simulink model "LMS_cs_2018"  (R2018a)
settings: Solver=ode5  StartTime=0.0  StopTime=inf  FixedStep=1/200  RelTol=1e-3
PreLoadFcn:
  | mbxruntime.callbacks.PreLoadFcn(bdroot);
PostLoadFcn:
  | mbxruntime.callbacks.PostLoadFcn(bdroot);
InitFcn:
  | mbxruntime.callbacks.InitFcn(bdroot);
StartFcn:
  | mbxruntime.callbacks.StartFcn(bdroot);
StopFcn:
  | mbxruntime.callbacks.StopFcn(bdroot);
model workspace (MAT data in the model file):
  mbox_table : struct (value not decoded)
  model_closed = 0
  sim_status = 0
undefined symbols (not defined in the file or in its folder): DiscIntNeverNeededParam, serial, WheelL0, WheelL1, WheelR0, WheelR1
libraries: simulink x298, simulink_extras x78, PreScanSimulinkLibrary x29, PreScanUsefulBlocks x6, instrumentlib x5, simulink_need_slupdate x1
(part 2 of 45)

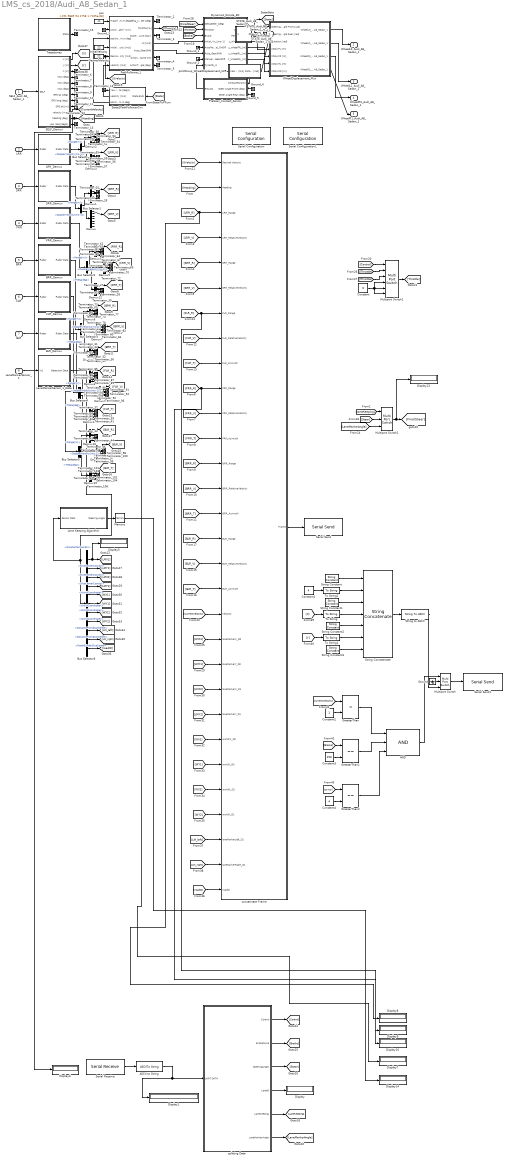
== system LMS_cs_2018/Audi_A8_Sedan_1 ==
  SELF_Audi_A8_Sedan_1 : Inport  Tag=inport/SelfPort  OutDataTypeStr=Bus: PRESCAN_SELFSENSORDATA  PortDimensions=1  SampleTime=2/200  BusOutputAsStruct=on
  LRR : Inport  Tag=inport/Radar  Port=2  OutDataTypeStr=Bus: PRESCAN_SCANNERSENSOR_MESSAGE  PortDimensions=7  SampleTime=1/4  BusOutputAsStruct=on
  SRR : Inport  Tag=inport/Radar  Port=3  OutDataTypeStr=Bus: PRESCAN_SCANNERSENSOR_MESSAGE  PortDimensions=7  SampleTime=1/4  BusOutputAsStruct=on
  FRR : Inport  Tag=inport/Radar  Port=4  OutDataTypeStr=Bus: PRESCAN_SCANNERSENSOR_MESSAGE  PortDimensions=7  SampleTime=1/4  BusOutputAsStruct=on
  BRR : Inport  Tag=inport/Radar  Port=5  OutDataTypeStr=Bus: PRESCAN_SCANNERSENSOR_MESSAGE  PortDimensions=7  SampleTime=1/4  BusOutputAsStruct=on
  FLR : Inport  Tag=inport/Radar  Port=6  OutDataTypeStr=Bus: PRESCAN_SCANNERSENSOR_MESSAGE  PortDimensions=7  SampleTime=1/4  BusOutputAsStruct=on
  BLR : Inport  Tag=inport/Radar  Port=7  OutDataTypeStr=Bus: PRESCAN_SCANNERSENSOR_MESSAGE  PortDimensions=7  SampleTime=1/4  BusOutputAsStruct=on
  LaneMarkerSensor_1 : Inport  Tag=inport/LaneMarker  Port=8  OutDataTypeStr=Bus: PRESCAN_LANEMARKER_MESSAGE  PortDimensions=2  SampleTime=1/20  BusOutputAsStruct=on
  AND : Logic  Inputs=3  IconShape=distinctive  AllPortsSameDT=off  OutDataTypeStr=boolean
  ASCII to String : ASCIIToString
  BLR_Demux : Subsystem  Tag=demux/Radar  TreatAsAtomicUnit=on  mask(PreScan Demux Block: Radar){MAXMESSAGES=7}
      mask prompts: MAXMESSAGES "Number of Objects"
      mask help:
      | The Radar Sensor is a detailed sensor based on a physical radar
      | model that includes Antenna GAIN Maps (AGM) and atmospheric
      | attenuation.
      |
      | For more information, please click Help.
      mask Help: eval('openHelp(1464)')
      mask Display:
      | port_label('input',1,'Radar')
      | port_label('output',1,'Radar Data')
  BRR_Demux : Subsystem  Tag=demux/Radar  TreatAsAtomicUnit=on  mask(PreScan Demux Block: Radar){MAXMESSAGES=7}
      mask prompts: MAXMESSAGES "Number of Objects"
      mask help:
      | The Radar Sensor is a detailed sensor based on a physical radar
      | model that includes Antenna GAIN Maps (AGM) and atmospheric
      | attenuation.
      |
      | For more information, please click Help.
      mask Help: eval('openHelp(1464)')
      mask Display:
      | port_label('input',1,'Radar')
      | port_label('output',1,'Radar Data')
  Bus Selector : BusSelector  OutputSignals=Range[m],DopplerVelocity[ms-1]
  Bus Selector1 : BusSelector  OutputSignals=Range[m],DopplerVelocity[ms-1]
  Bus Selector{2..5} (4 alike) : BusSelector  OutputSignals=Range[m],DopplerVelocity[ms-1],Theta[deg]
  Bus Selector6 : BusSelector  OutputSignals=ScanAtSensor.SliceCenterCoordsX,ScanAtSensor.SliceCenterCoordsY,ScanAtDistance1.SliceCenterCoordsX,ScanAtDistance1.SliceCenterCoordsY,ScanAtSensor.RightLaneIntersection1.WorldCoordinateX,ScanAtSensor.RightLaneIntersection1.WorldCoordinateY,ScanAtDistance1.RightLaneIntersection1.WorldCoordinateX,ScanAtDistance1.RightLaneIntersection1.WorldCoordinateY,ScanAtDistance1.LeftLaneIntersection1.DistanceFromScanCenter,ScanAtDistance1.RightLaneIntersection1.DistanceFromScanCenter,ScanAtDistance1.RoadIdUnderSliceCenter
  Constant : Constant  Value=0
  Constant1 : Constant  Value=4
  Constant2 : Constant
  Constant3 : Constant  Value=150
  Constant4 : Constant  Value=4
  Demux{,1..15} (16 alike) : Demux  Outputs=7
  DesiredVelocity : Constant  Tag=DesiredVelocity  Value=22
  Display{,1,5..10,13..14} (10 alike) : Display
  Dynamics_Simple_3D : Subsystem  Tag=Simple_Vehicle_Dynamics_3D  mask(PreScan Block: Simple Dynamics 3D){Migrate=on, TimeStep=1/200, ComputationMode=Continuous_Time}
      mask prompts: Migrate "Migrate. During migration this block will be replaced by a newer one."; TimeStep "Auto assigned: Time Step [s]"; ComputationMode "Computation mode:"
      mask help:
      | The Simple Dynamics Model is selected in the GUI to simulate vehicle dynamics behavior.
      |
      | The Simple Dynamics Model is completely open to the user. The parameters of this model can be set in the Simple Dynamics dialog in the GUI.
      |
      | For more information, please click Help.
      mask init:
      | p = SimpleDyn_pars;
      settings: DeleteFcn=PreScanBlockDeleteFcn;
      mask Help: eval('openHelp(260)')
      mask Display:
      | image(imread('SimpleDyn.png'))
      | port_label('input', 1, '{\delta}_S_t_ _e_e_r [deg]','texmode','on')
      | port_label('input', 2, 'Throttle [%]')
      | port_label('input', 3, 'Brake Pres [bar]')
      | port_label('input', 4, 'V_0 [ms-1]','texmode','on')
      | port_label('input', 5, 'Auto=[0]/Manual=[1]')
      | port_label('input', 6, 'Auto_GearShift')
      | port_label('input', 7, 'Manual_GearShift')
      | port_label('input', 8, 'TyreInfo_in')
      | port_label('output', 1, 'State')
      | port_label('output', 2, 'Vx [ms-1]')
      | port_label('output', 3, 'Perf Params')
      | port_label('output', 4, 'zDispFL[m]')
      | port_label('output', 5, 'zDispFR[m]')
      | port_label('output', 6, 'zDispRL[m]')
      | port_label('output', 7, 'zDispRR[m]')
  FLR_Demux : Subsystem  Tag=demux/Radar  TreatAsAtomicUnit=on  mask(PreScan Demux Block: Radar){MAXMESSAGES=7}
      mask prompts: MAXMESSAGES "Number of Objects"
      mask help:
      | The Radar Sensor is a detailed sensor based on a physical radar
      | model that includes Antenna GAIN Maps (AGM) and atmospheric
      | attenuation.
      |
      | For more information, please click Help.
      mask Help: eval('openHelp(1464)')
      mask Display:
      | port_label('input',1,'Radar')
      | port_label('output',1,'Radar Data')
  FRR_Demux : Subsystem  Tag=demux/Radar  TreatAsAtomicUnit=on  mask(PreScan Demux Block: Radar){MAXMESSAGES=7}
      mask prompts: MAXMESSAGES "Number of Objects"
      mask help:
      | The Radar Sensor is a detailed sensor based on a physical radar
      | model that includes Antenna GAIN Maps (AGM) and atmospheric
      | attenuation.
      |
      | For more information, please click Help.
      mask Help: eval('openHelp(1464)')
      mask Display:
      | port_label('input',1,'Radar')
      | port_label('output',1,'Radar Data')
  GreaterThan : RelationalOperator  Operator=<  OutDataTypeStr=boolean  RndMeth=Simplest
  GreaterThan1 : RelationalOperator  Operator===  OutDataTypeStr=boolean  RndMeth=Simplest
  GreaterThan2 : RelationalOperator  Operator===  OutDataTypeStr=boolean  RndMeth=Simplest
  Ground : Ground
  Ground_{1..7} (7 alike) : Ground
  InitialVelocity : Constant  Tag=InitialVelocity  Value=22
  JointGroup_WheelDisplacement_V2R : Subsystem  Tag=mux/Wheels  mask(PreScan Velocity to Wheel Angle Block:){TimeStep=2/200, TireRadius=0.34}
      mask prompts: TimeStep "Auto Assigned: Time Step [s]"; TireRadius "Tire Radius [m]"
      settings: DeleteFcn=PreScanBlockDeleteFcn;
      mask Display: disp('Velocity\nto\nWheelAngle')
  LRR_Demux : Subsystem  Tag=demux/Radar  TreatAsAtomicUnit=on  mask(PreScan Demux Block: Radar){MAXMESSAGES=7}
      mask prompts: MAXMESSAGES "Number of Objects"
      mask help:
      | The Radar Sensor is a detailed sensor based on a physical radar
      | model that includes Antenna GAIN Maps (AGM) and atmospheric
      | attenuation.
      |
      | For more information, please click Help.
      mask Help: eval('openHelp(1464)')
      mask Display:
      | port_label('input',1,'Radar')
      | port_label('output',1,'Radar Data')
  Lane Keeping Algorithm : Subsystem
  LaneMarkerSensor_1_Data : Subsystem  Tag=demux/LaneMarkerSensor  mask{NUMBEROFSLICES=2, TimeStep=1/20}
      mask prompts: NUMBEROFSLICES "Number of slices"; TimeStep "Auto Assigned: Time Step [s]"
      mask Help: eval('openHelp(2301)')
  Memory : Memory
  Multiport Switch : MultiPortSwitch  DataPortOrder=Zero-based contiguous  Inputs=2  zeroidx=on
  Multiport Switch1 : MultiPortSwitch  DataPortOrder=Zero-based contiguous  Inputs=5  zeroidx=on
  Multiport Switch2 : MultiPortSwitch  DataPortOrder=Zero-based contiguous  Inputs=2  zeroidx=on
  PathFollower_1 : Subsystem  Tag=pathFollower  mask(PreScan Block: Path Follower){Migrate=on, FileName='Trajectory_1.mat', TunableSteeringGain=1, XShifting_wrt_COG=0}
      mask prompts: Migrate "Migrate. During migration this block will be replaced by a newer one."; FileName "Trajectory Name"; TunableSteeringGain "TunableSteeringGain [-]"; XShifting_wrt_COG "XShifting_wrt_COG [m]"
      mask help:
      | The Path Follower Model is selected in the GUI to simulate driver behavior.
      |
      | For more information, please click Help.
      mask init:
      | load(['trajectories/',eval(FileName)])
      | traject=trajectory';
      | 
      | Traj_x=traject(:,2);
      | Traj_y=traject(:,3);
      | Traj_z=traject(:,4);
      | Traj_vx=traject(:,8);
      | Traj_vy=traject(:,9);
      | Traj_vz=traject(:,10);
      mask Help: eval('openHelp(232)')
  PreScan_Contact_Sensor : Subsystem  Tag=PreScan_Contact_Sensor  LoadFcn=|  mask(PreScan Block: PreScan Contact Sensor){x0=-191.9885, y0=94.1758, z0=0.55, Roll0=0, Pitch0=0, Yaw0=1.7105e-08, wheelRadius=0.34, hcog=0.55, b=1.77, TimeStep=1/200}
      | load PrescanXYZData;
      | load PrescanRPYData;
      | load PrescanQuatData;
      | load PrescanAxisAngleData;
      | load PrescanPoseData;
      | load PrescanPoseQData;
      | load PrescanPoseAData;
      | load PrescanWheelContactData;
      mask prompts: x0 "Ini x-position VEHICLE wrt GLOBAL axis system [m]"; y0 "Ini y-position VEHICLE wrt GLOBAL axis system [m]"; z0 "Ini z-position VEHICLE wrt GLOBAL axis system [m]"; Roll0 "Ini roll-angle BODY wrt VEHICLE axis system [deg]"; Pitch0 "Ini pitch-angle BODY wrt VEHICLE axis system [deg]"; Yaw0 "Ini yaw-angle VEHICLE wrt GLOBAL axis system [deg]"; wheelRadius "Wheel Radius [m]"; hcog "Dynamics: hCoG [m]"; b "Dynamics: b [m]"; TimeStep "Time Step [s]"
      mask help:
      | This block encapsulates the base Contact sensor.
      |
      | It takes input parameters from the PreScan 3D vehicle dynamics block and outputs contact results.
      mask Help: eval('openHelp(251)')
  SELF_Demux : Subsystem  Tag=demux/SelfPort  mask(PreScan Demux Block:){}
      mask help:
      | The SELF port shows (state) information of the actor itself. The outputs are position in the experiment's axis system and the GPS coordinates, and the object's absolute velocity and compass heading.
      |
      | For more information, please click Help.
      settings: DeleteFcn=PreScanBlockDeleteFcn;
      mask Help: eval('openHelp(462)')
      mask Display:
      | port_label('output',1,'x [m]')
      | port_label('output',2,'y [m]')
      | port_label('output',3,'z [m]','texmode','on')
      | port_label('output',4,'Rotx [deg]','texmode','on')
      | port_label('output',5,'Roty [deg]','texmode','on')
      | port_label('output',6,'Rotz [deg]','texmode','on')
      | port_label('output',7,'GPS lat [deg]','texmode','on')
      | port_label('output',8,'GPS long [deg]','texmode','on')
      | port_label('output',9,'GPS alt [m]','texmode','on')
      | port_label('output',10,'Velocity [m/s]')
      | port_label('output',11,'Heading [deg]')
      | port_label('output',12,'Yaw rate [deg/s]')
  SRR_Demux : Subsystem  Tag=demux/Radar  TreatAsAtomicUnit=on  mask(PreScan Demux Block: Radar){MAXMESSAGES=7}
      mask prompts: MAXMESSAGES "Number of Objects"
      mask help:
      | The Radar Sensor is a detailed sensor based on a physical radar
      | model that includes Antenna GAIN Maps (AGM) and atmospheric
      | attenuation.
      |
      | For more information, please click Help.
      mask Help: eval('openHelp(1464)')
      mask Display:
      | port_label('input',1,'Radar')
      | port_label('output',1,'Radar Data')
  STATE_Audi_A8_Sedan_1 : Subsystem  Tag=mux/StatePort  Priority=0  LoadFcn=load PrescanStateActuatorData  mask(PreScan Sink Block: State){x0=-191.9885, y0=94.1758, z0=0.55, Roll0=0, Pitch0=0, Yaw0=1.7105e-08, TimeStep=1/200}
      mask prompts: x0 "Ini x-position VEHICLE wrt GLOBAL axis system [m]"; y0 "Ini y-position VEHICLE wrt GLOBAL axis system [m]"; z0 "Ini z-position VEHICLE wrt GLOBAL axis system [m]"; Roll0 "Ini roll-angle BODY wrt VEHICLE axis system [deg]"; Pitch0 "Ini pitch-angle BODY wrt VEHICLE axis system [deg]"; Yaw0 "Ini yaw-angle VEHICLE wrt GLOBAL axis system [deg]"; TimeStep "Auto-Assigned: Upload Period [s]"
      mask help:
      | The Actor State contains a vector signal of size (9x1), containing the following signals:
      |
      | -  Position                  (x,y,z)                                     [m]
      | -  Velocity                  (vx,vy,vz)                               [m/s]
      | -  Angles                    (Roll, Pitch, Yaw)                   [rad]
      |
      | The Actor state is defined in the global axis system.
      | The state is superponed on the Initial position defined in the GUI.
      |
      | For more information, please click Help.
      settings: DeleteFcn=PreScanBlockDeleteFcn;
      mask Help: eval('openHelp(222)')
      mask Display: image(imread('State.png'))
  STATE_Audi_A8_Sedan_1_rc : RateTransition  Tag=mux_rc/StatePort  OutPortSampleTimeOpt=Inherit
  Serial Receive : instrumentlib/Serial Receive  Priority=1  ObjConstructor=serial('COM5');  ComPortMenu=COM5  ComPort=COM5  DataType=uint8  DataSize="[1  21]"  EnableBlockingMode=on  ActionDataUnavailable=Output last received value  CustomValue=0  SampleTime=0.005
  Serial Configuration : instrumentlib/Serial Configuration  Priority=-200000  ObjConstructor=serial('COM5');  ComPortMenu=COM5  ComPort=COM5  BaudRate=115200  DataBits=8  Parity=none  StopBits=1  ByteOrder=LittleEndian  FlowControl=none  Timeout=0.001
  Serial Configuration1 : instrumentlib/Serial Configuration  Priority=-200000  PortSel=COM6  Port=COM6  ComPort=COM6  BaudRate=115200  DataBits=8  Parity=none  StopBits=1  ByteOrder=little-endian  FlowControl=none  Timeout=0.001  SimulateUsing=Interpreted execution  BlockInModel=on  aMode=1
  Serial Send : instrumentlib/Serial Send  Priority=1  ObjConstructor=serial('COM5');  ComPortMenu=COM5  ComPort=COM5  Terminator=<none>  EnableBlockingMode=on
  Serial Send1 : instrumentlib/Serial Send  Priority=1  PortSel=COM6  Port=COM6  ComPort=COM6  Header=[]  Terminator=<none>  CustomTerminator=[]  EnableBlockingMode=on  SimulateUsing=Interpreted execution  BlockInModel=on  aMode=1
  State2PathFollowerCnv : Subsystem  Tag=State2PFConnection/cnv
  String Concatenate : StringConcatenate  Inputs=7
  String Constant : StringConstant  String="\"*\""
  String Constant1 : StringConstant  String="\";\""
  String Constant2 : StringConstant  String="\"/\""
  String Constant3 : StringConstant  String="\"#\""
  String to ASCII : StringToASCII  MaximumLength=30
  Terminator_{1..15,24..106} (98 alike) : Terminator
  To String : ToString
  To String1 : ToString
  To String2 : ToString
  Trajectories : Subsystem  Tag=Trajectories  mask(PreScan Source Block: Trajectories){}
      mask help:
      | The Trajectory block contains the trajectories defined in the PreScan Experiment Editor. The output of the trajectory block is the (vehicle) State.
      |
      | For more information, please click Help.
      settings: DeleteFcn=PreScanBlockDeleteFcn;
      mask Help: eval('openHelp(312)')
      mask Display: image(imread('Trajectory.png'));
  WheelDisplacement_Mux : Subsystem  Tag=mux/JointGroup  mask(JointGroup){}
      mask help:
      | The JointGroup allows to control several Joints in one go, as defined for this particular model.
      | For more information, look in the PreScan manual in the section "Model Preparation Tool" -> "Joint Groups"
      |
      | For more information on the Joints simulink interface, press Help.
      mask Help: eval('openHelp(254)')
  concatinate Frame : Subsystem
  pos : Constant  Tag=pos  Value=[-191.9885 94.1758 1.7105e-08]
  splitting Data : Subsystem
  STATE_Audi_A8_Sedan_1_bus : Outport  Tag=outport/StatePort  OutDataTypeStr=Bus: PRESCAN_STATEACTUATORDATA  PortDimensions=1  SampleTime=2/200
  WheelL0_Audi_A8_Sedan_1 : Outport  Tag=outport/JointActuator  Port=2  OutDataTypeStr=Bus: PRESCAN_POSE_DATA  SampleTime=2/200
  WheelL1_Audi_A8_Sedan_1 : Outport  Tag=outport/JointActuator  Port=3  OutDataTypeStr=Bus: PRESCAN_POSE_DATA  SampleTime=2/200
  WheelR0_Audi_A8_Sedan_1 : Outport  Tag=outport/JointActuator  Port=4  OutDataTypeStr=Bus: PRESCAN_POSE_DATA  SampleTime=2/200
  WheelR1_Audi_A8_Sedan_1 : Outport  Tag=outport/JointActuator  Port=5  OutDataTypeStr=Bus: PRESCAN_POSE_DATA  SampleTime=2/200
  wires:
  Lane Keeping Algorithm/1(Steering Angle) -> Memory/1
  Demux2/5 -> Terminator_52/1
  Bus Selector/1 -> Demux2/1  "<Range[m]>"
  Demux3/4 -> Terminator_57/1
  Demux2/7 -> Terminator_54/1
  Demux2/4 -> Terminator_51/1
  Demux3/6 -> Terminator_59/1
  Demux3/7 -> Terminator_60/1
  Demux3/3 -> Terminator_56/1
  Demux2/3 -> Terminator_50/1
  Demux2/2 -> Terminator_49/1
  Demux2/6 -> Terminator_53/1
  Demux2/1 -> [LRR_R]
  Bus Selector/2 -> Demux3/1  "<DopplerVelocity[ms-1]>"
  Demux3/1 -> [LRR_V]
  Demux3/5 -> Terminator_58/1
  Demux3/2 -> Terminator_55/1
  LRR_Demux/1(Radar Data) -> Bus Selector/1
  Demux/3 -> ?
  Demux/2 -> ?
  Demux/4 -> ?
  Demux/5 -> ?
  Demux/6 -> ?
  Demux/7 -> ?
  Demux1/2 -> ?
  Demux1/4 -> Terminator_26/1
  Demux1/7 -> Terminator_24/1
  Bus Selector1/1 -> Demux1/1  "<Range[m]>"
  Bus Selector1/2 -> Demux/1  "<DopplerVelocity[ms-1]>"
  Demux1/3 -> Terminator_25/1
  Demux/1 -> [SRR_V]
  Demux1/1 -> [SRR_R]
  Demux1/6 -> ?
  Demux1/5 -> ?
  SRR_Demux/1(Radar Data) -> Bus Selector1/1
  Demux12/4 -> Terminator_27/1
  Demux4/2 -> Terminator_61/1
  Demux5/2 -> Terminator_67/1
  Demux12/6 -> Terminator_29/1
  Demux4/6 -> Terminator_65/1
  Demux5/5 -> Terminator_70/1
  Demux12/2 -> ?
  Demux5/6 -> Terminator_71/1
  Demux5/4 -> Terminator_69/1
  Demux4/1 -> [FRR_R]
  Demux4/4 -> Terminator_63/1
  Demux4/7 -> Terminator_66/1
  Demux12/1 -> [FRR_T]
  Demux4/3 -> Terminator_62/1
  Demux12/7 -> Terminator_30/1
  Demux4/5 -> Terminator_64/1
  Demux12/3 -> ?
  Demux5/7 -> Terminator_72/1
  Demux5/3 -> Terminator_68/1
  Demux5/1 -> [FRR_V]
  Demux12/5 -> Terminator_28/1
  Bus Selector2/3 -> Demux12/1  "<Theta[deg]>"
  Bus Selector2/1 -> Demux4/1  "<Range[m]>"
  Bus Selector2/2 -> Demux5/1  "<DopplerVelocity[ms-1]>"
  FRR_Demux/1(Radar Data) -> Bus Selector2/1
  Demux13/4 -> Terminator_33/1
  Bus Selector3/3 -> Demux13/1  "<Theta[deg]>"
  Demux7/7 -> Terminator_84/1
  Demux13/5 -> Terminator_34/1
  Demux7/3 -> Terminator_80/1
  Demux6/3 -> Terminator_74/1
  Demux13/3 -> Terminator_32/1
  Demux7/6 -> Terminator_83/1
  Demux6/2 -> Terminator_73/1
  Demux7/4 -> Terminator_81/1
  Demux7/5 -> Terminator_82/1
  Demux7/2 -> Terminator_79/1
  Demux6/4 -> Terminator_75/1
  Demux6/6 -> Terminator_77/1
  Demux6/5 -> Terminator_76/1
  Demux6/1 -> [BRR_R]
  Demux7/1 -> [BRR_V]
  Bus Selector3/1 -> Demux6/1  "<Range[m]>"
  Demux13/6 -> Terminator_35/1
  Bus Selector3/2 -> Demux7/1  "<DopplerVelocity[ms-1]>"
  Demux13/2 -> Terminator_31/1
  Demux13/7 -> Terminator_36/1
  Demux6/7 -> Terminator_78/1
  Demux13/1 -> [BRR_T]
  BRR_Demux/1(Radar Data) -> Bus Selector3/1
  Demux14/4 -> Terminator_39/1
  Demux14/5 -> Terminator_40/1
  Bus Selector4/2 -> Demux9/1  "<DopplerVelocity[ms-1]>"
  Demux9/7 -> Terminator_96/1
  Demux8/3 -> Terminator_86/1
  Demux8/5 -> Terminator_88/1
  Demux9/4 -> Terminator_93/1
  Demux8/6 -> Terminator_89/1
  Demux8/4 -> Terminator_87/1
  Demux8/7 -> Terminator_90/1
  Demux8/2 -> Terminator_85/1
  Demux8/1 -> [FLR_R]
  Demux14/2 -> Terminator_37/1
  Demux14/6 -> Terminator_41/1
  Demux9/3 -> Terminator_92/1
  Demux9/2 -> Terminator_91/1
  Demux9/1 -> [FLR_V]
  Demux9/5 -> Terminator_94/1
  Demux14/3 -> Terminator_38/1
  Bus Selector4/1 -> Demux8/1  "<Range[m]>"
  Demux9/6 -> Terminator_95/1
  Bus Selector4/3 -> Demux14/1  "<Theta[deg]>"
  Demux14/7 -> Terminator_42/1
  Demux14/1 -> [FLR_T]
  FLR_Demux/1(Radar Data) -> Bus Selector4/1
  Demux15/6 -> Terminator_105/1
  Demux15/3 -> Terminator_102/1
  Demux15/1 -> [BLR_T]
  Demux10/3 -> ?
  Demux15/2 -> Terminator_101/1
  Demux11/2 -> Terminator_47/1
  Demux11/7 -> Terminator_100/1
  Demux11/5 -> Terminator_98/1
  Demux11/6 -> Terminator_99/1
  Demux11/4 -> Terminator_97/1
  Demux15/5 -> Terminator_104/1
  Demux15/4 -> Terminator_103/1
  Demux10/4 -> Terminator_43/1
  Demux10/2 -> ?
  Demux11/3 -> Terminator_48/1
  Bus Selector5/1 -> Demux10/1  "<Range[m]>"
  Demux15/7 -> Terminator_106/1
  Demux10/1 -> [BLR_R]
  Demux10/6 -> Terminator_45/1
  Demux11/1 -> [BLR_V]
  Bus Selector5/2 -> Demux11/1  "<DopplerVelocity[ms-1]>"
  Bus Selector5/3 -> Demux15/1  "<Theta[deg]>"
  Demux10/7 -> Terminator_46/1
  Demux10/5 -> Terminator_44/1
  BLR_Demux/1(Radar Data) -> Bus Selector5/1
  [FLR_R] -> Display10/1, concatinate Frame/7(" FLR_Range")
  [SRR_R] -> concatinate Frame/5(" SRR_Range")
  [LRR_V] -> concatinate Frame/4(LRR_RelativeVelocity)
  [BLR_T] -> concatinate Frame/18(" BLR_Azimuth")
  [FRR_R] -> Display9/1, concatinate Frame/10(" FRR_Range")
  [BRR_T] -> concatinate Frame/15(" BRR_Azimuth")
  [FLR_T] -> concatinate Frame/9(FLR_Azimuth)
  [FRR_T] -> concatinate Frame/12(" FRR_Azimuth")
  [FRR_V] -> concatinate Frame/11(" FRR_RelativeVelocity")
  [LRR_R] -> Display8/1, concatinate Frame/3(" LRR_Range")
  [FLR_V] -> concatinate Frame/8(" FLR_RelativeVelocity")
  concatinate Frame/1(Frame) -> Serial Send/1
  [BLR_V] -> concatinate Frame/17(" BLR_RelativeVelocity")
  [BRR_V] -> concatinate Frame/14(" BRR_RelativeVelocity")
  [SRR_V] -> concatinate Frame/6(" SRR_RelativeVelocity")
  [BLR_R] -> concatinate Frame/16(" BLR_Range")
  [Heading] -> concatinate Frame/2(Heading)
  [BRR_R] -> concatinate Frame/13(" BRR_Range")
  splitting Data/1(Control) -> [Control]
  Serial Receive/1 -> ASCII to String/1
  ASCII to String/1 -> splitting Data/1(UART DATA), Display1/1
  splitting Data/2(BrakeForce) -> [Brake]
  splitting Data/4(LaneID) -> Display/1
  splitting Data/3(SteeringAngle) -> [Steer]
  Constant/1 -> Multiport Switch1/6, Multiport Switch1/4, Multiport Switch1/5
  [IThrottle] -> Multiport Switch1/3
  [Control] -> Multiport Switch1/1
  [IThrottle] -> Multiport Switch1/2
  Multiport Switch1/1 -> [Throttle]
  SELF_Demux/11(heading [deg]) -> Display7/1, [Heading]
  PathFollower_1/2(throttle [%]) -> [IThrottle]
  [Throttle] -> Dynamics_Simple_3D/2(Throttle)
  [Brake] -> Dynamics_Simple_3D/3(Brake)
  PathFollower_1/4(v0 [m/s]) -> Dynamics_Simple_3D/4(Initial_Vx_[ms-1])
  Multiport Switch2/1 -> Display13/1, [FinalSteer]
  SELF_Demux/10(velocity [m/s]) -> Display6/1, [CurrentVelocity]
  [FinalSteer] -> Dynamics_Simple_3D/1(DeltaSteer_[deg])
  [LaneKeeping] -> Multiport Switch2/1
  [Steer] -> Multiport Switch2/2
  splitting Data/5(LaneKeeping) -> [LaneKeeping]
  [DVelocity] -> concatinate Frame/1(" Desired Velocity")
  [CurrentVelocity] -> concatinate Frame/19(Velocity)
  splitting Data/6(LaneMarkerAngle) -> [LaneMarkerAngle]
  LaneMarkerSensor_1_Data/1(Detection Data) -> Bus Selector6/1, Lane Keeping Algorithm/1(Sensor Data)
  Bus Selector6/1 -> Display5/1, [LMX1]  "<SliceCenterCoordsX>"
  Bus Selector6/2 -> [LMY1]  "<SliceCenterCoordsY>"
  Bus Selector6/3 -> [LMX2]  "<SliceCenterCoordsX>"
  Bus Selector6/4 -> [LMY2]  "<SliceCenterCoordsY>"
  Bus Selector6/5 -> [WX1]  "<WorldCoordinateX>"
  Bus Selector6/6 -> [WY1]  "<WorldCoordinateY>"
  Bus Selector6/7 -> [WX2]  "<WorldCoordinateX>"
  Bus Selector6/8 -> [WY2]  "<WorldCoordinateY>"
  Bus Selector6/11 -> [roadID]  "<RoadIdUnderSliceCenter>"
  [LMX1] -> concatinate Frame/20(laneMarkerX_D0)
  [LMY1] -> concatinate Frame/21(laneMarkerY_D0)
  [LMX2] -> concatinate Frame/22(laneMarkerX_D1)
  [LMY2] -> concatinate Frame/23(laneMarkerY_D1)
  [WX2] -> concatinate Frame/26(worldX_D1)
  [WY1] -> concatinate Frame/25(worldY_D0)
  [WX1] -> concatinate Frame/24(worldrX_D0)
  [WY2] -> concatinate Frame/27(worldY_D1)
  [roadID] -> concatinate Frame/30(roadID)
  [LM_left] -> concatinate Frame/28(laneMarkerLeft_D1)
  [LM_right] -> concatinate Frame/29(laneMarkerRight_D1)
  Bus Selector6/9 -> [LM_left]  "<DistanceFromScanCenter>"
  Bus Selector6/10 -> [LM_right]  "<DistanceFromScanCenter>"
  Memory/1 -> Display14/1
  [LaneMarkerAngle] -> Multiport Switch2/3
  DesiredVelocity/1 -> [DVelocity], PathFollower_1/5(Desired Velocity [m/s])
  SELF_Demux/1(x [m]) -> [X]
  SELF_Demux/2(y [m]) -> [Y]
  [X] -> To String/1
  [Y] -> To String1/1
  Constant1/1 -> To String2/1
  To String2/1 -> String Concatenate/2
  To String/1 -> String Concatenate/4
  To String1/1 -> String Concatenate/6
  String Constant/1 -> String Concatenate/1
  String Constant1/1 -> String Concatenate/3
  String Constant2/1 -> String Concatenate/5
  String Constant3/1 -> String Concatenate/7
  String Concatenate/1 -> String to ASCII/1
  STATE_Audi_A8_Sedan_1_rc/1 -> STATE_Audi_A8_Sedan_1_bus/1
  STATE_Audi_A8_Sedan_1/1(StateBus) -> STATE_Audi_A8_Sedan_1_rc/1, [State]
  SELF_Audi_A8_Sedan_1/1 -> SELF_Demux/1(SELF)
  LRR/1 -> LRR_Demux/1(Radar)
  SRR/1 -> SRR_Demux/1(Radar)
  FRR/1 -> FRR_Demux/1(Radar)
  BRR/1 -> BRR_Demux/1(Radar)
  FLR/1 -> FLR_Demux/1(Radar)
  BLR/1 -> BLR_Demux/1(Radar)
  LaneMarkerSensor_1/1 -> LaneMarkerSensor_1_Data/1(In1)
  WheelDisplacement_Mux/1(WheelL0_Audi_A8_Sedan_1) -> WheelL0_Audi_A8_Sedan_1/1
  WheelDisplacement_Mux/2(WheelL1_Audi_A8_Sedan_1) -> WheelL1_Audi_A8_Sedan_1/1
  WheelDisplacement_Mux/3(WheelR0_Audi_A8_Sedan_1) -> WheelR0_Audi_A8_Sedan_1/1
  WheelDisplacement_Mux/4(WheelR1_Audi_A8_Sedan_1) -> WheelR1_Audi_A8_Sedan_1/1
  JointGroup_WheelDisplacement_V2R/1(Rotation [rad]) -> WheelDisplacement_Mux/3(Rotation [rad])
  Dynamics_Simple_3D/8(ContactParams) -> PreScan_Contact_Sensor/1(ContactParams)
  PreScan_Contact_Sensor/1(Results) -> Dynamics_Simple_3D/8(TyreInfo_in)
  Dynamics_Simple_3D/2(Vx [m s-1]) -> JointGroup_WheelDisplacement_V2R/1(Velocity [m/s])
  Dynamics_Simple_3D/4(z_wheelFL_[m]) -> WheelDisplacement_Mux/4(zDisp FL [m])
  Dynamics_Simple_3D/5(z_wheelFR_[m]) -> WheelDisplacement_Mux/5(zDisp FR [m])
  Dynamics_Simple_3D/6(z_wheelRL_[m]) -> WheelDisplacement_Mux/6(zDisp RL [m])
  Dynamics_Simple_3D/7(z_wheelRR_[m]) -> WheelDisplacement_Mux/7(zDisp RR [m])
  pos/1 -> PathFollower_1/1(TrajOffset_x,y,Y [m,m,deg])
  InitialVelocity/1 -> PathFollower_1/4(Initial Velocity [m/s])
  [State] -> State2PathFollowerCnv/1(State BUS)
  State2PathFollowerCnv/2(velocity [m/s]) -> PathFollower_1/6(velocity [m/s])
  State2PathFollowerCnv/3(position x,y,Y [m,m,deg]) -> PathFollower_1/3(position x,y,Y [m,m,deg])
  PathFollower_1/5(Auto_GearShift) -> Dynamics_Simple_3D/6(Auto_GearShift)
  Dynamics_Simple_3D/1(State) -> STATE_Audi_A8_Sedan_1/1(State)
  Ground_1/1 -> Dynamics_Simple_3D/5(AutoManual_OnOff)
  Ground_2/1 -> Dynamics_Simple_3D/7(Manual_GearShift)
  Dynamics_Simple_3D/3(Perf_Params) -> Terminator_1/1
  Ground_3/1 -> PathFollower_1/2(ActorOffset_Left(+) / Right(-) [m])
  PathFollower_1/1(delta_steerwheel [deg]) -> Terminator_2/1
  PathFollower_1/3(brake pressure [bar]) -> Terminator_3/1
  PathFollower_1/6(Actor/Traj_distance [m]) -> Terminator_4/1
  PathFollower_1/7(Actor/Traj_angle [deg]) -> Terminator_5/1
  Ground_4/1 -> PreScan_Contact_Sensor/2(Steer Angle Front [deg])
  Ground_5/1 -> PreScan_Contact_Sensor/3(Steer Angle Rear [deg])
  SELF_Demux/3(z [m]) -> Terminator_6/1
  SELF_Demux/4(rotx [deg]) -> Terminator_7/1
  SELF_Demux/5(roty [deg]) -> Terminator_8/1
  SELF_Demux/6(rotz [deg]) -> Terminator_9/1
  SELF_Demux/7(GPS lat [deg]) -> Terminator_10/1
  SELF_Demux/8(GPS long [deg]) -> Terminator_11/1
  SELF_Demux/9(GPS alt [m]) -> Terminator_12/1
  SELF_Demux/12(yaw rate [deg/s]) -> Terminator_13/1
  State2PathFollowerCnv/1(Yaw rate [deg/s]) -> Terminator_14/1
  Trajectories/1(State) -> Terminator_15/1
  Ground_6/1 -> WheelDisplacement_Mux/1(Steering Angle Front [rad])
  Ground_7/1 -> WheelDisplacement_Mux/2(Steering Angle Rear [rad])
  Constant2/1 -> GreaterThan/2
  [CurrentVelocity] -> GreaterThan/1
  GreaterThan/1 -> AND/1
  Constant3/1 -> GreaterThan1/2
  [Brake] -> GreaterThan1/1
  GreaterThan1/1 -> AND/2
  Multiport Switch/1 -> Serial Send1/1
  AND/1 -> Multiport Switch/1
  String to ASCII/1 -> Multiport Switch/3
  Ground/1 -> Multiport Switch/2
  [Control] -> GreaterThan2/1
  Constant4/1 -> GreaterThan2/2
  GreaterThan2/1 -> AND/3

== system LMS_cs_2018/Audi_A8_Sedan_2 ==
  SELF_Audi_A8_Sedan_2 : Inport  Tag=inport/SelfPort  OutDataTypeStr=Bus: PRESCAN_SELFSENSORDATA  PortDimensions=1  SampleTime=2/200  BusOutputAsStruct=on
  Auto_Gear : Constant  Tag=AutoGear
  Dynamics_Simple_3D : Subsystem  Tag=Simple_Vehicle_Dynamics_3D  mask(PreScan Block: Simple Dynamics 3D){Migrate=on, TimeStep=1/200, ComputationMode=Continuous_Time}
      mask prompts: Migrate "Migrate. During migration this block will be replaced by a newer one."; TimeStep "Auto assigned: Time Step [s]"; ComputationMode "Computation mode:"
      mask help:
      | The Simple Dynamics Model is selected in the GUI to simulate vehicle dynamics behavior.
      |
      | The Simple Dynamics Model is completely open to the user. The parameters of this model can be set in the Simple Dynamics dialog in the GUI.
      |
      | For more information, please click Help.
      mask init:
      | p = SimpleDyn_pars;
      settings: DeleteFcn=PreScanBlockDeleteFcn;
      mask Help: eval('openHelp(260)')
      mask Display:
      | image(imread('SimpleDyn.png'))
      | port_label('input', 1, '{\delta}_S_t_ _e_e_r [deg]','texmode','on')
      | port_label('input', 2, 'Throttle [%]')
      | port_label('input', 3, 'Brake Pres [bar]')
      | port_label('input', 4, 'V_0 [ms-1]','texmode','on')
      | port_label('input', 5, 'Auto=[0]/Manual=[1]')
      | port_label('input', 6, 'Auto_GearShift')
      | port_label('input', 7, 'Manual_GearShift')
      | port_label('input', 8, 'TyreInfo_in')
      | port_label('output', 1, 'State')
      | port_label('output', 2, 'Vx [ms-1]')
      | port_label('output', 3, 'Perf Params')
      | port_label('output', 4, 'zDispFL[m]')
      | port_label('output', 5, 'zDispFR[m]')
      | port_label('output', 6, 'zDispRL[m]')
      | port_label('output', 7, 'zDispRR[m]')
  Ground_{1..10} (10 alike) : Ground
  JointGroup_WheelDisplacement_V2R : Subsystem  Tag=mux/Wheels  mask(PreScan Velocity to Wheel Angle Block:){TimeStep=2/200, TireRadius=0.34}
      mask prompts: TimeStep "Auto Assigned: Time Step [s]"; TireRadius "Tire Radius [m]"
      settings: DeleteFcn=PreScanBlockDeleteFcn;
      mask Display: disp('Velocity\nto\nWheelAngle')
  PreScan_Contact_Sensor : Subsystem  Tag=PreScan_Contact_Sensor  LoadFcn=|  mask(PreScan Block: PreScan Contact Sensor){x0=62.0152, y0=90.3976, z0=0.55, Roll0=0, Pitch0=0, Yaw0=0, wheelRadius=0.34, hcog=0.55, b=1.77, TimeStep=1/200}
      | load PrescanXYZData;
      | load PrescanRPYData;
      | load PrescanQuatData;
      | load PrescanAxisAngleData;
      | load PrescanPoseData;
      | load PrescanPoseQData;
      | load PrescanPoseAData;
      | load PrescanWheelContactData;
      mask prompts: x0 "Ini x-position VEHICLE wrt GLOBAL axis system [m]"; y0 "Ini y-position VEHICLE wrt GLOBAL axis system [m]"; z0 "Ini z-position VEHICLE wrt GLOBAL axis system [m]"; Roll0 "Ini roll-angle BODY wrt VEHICLE axis system [deg]"; Pitch0 "Ini pitch-angle BODY wrt VEHICLE axis system [deg]"; Yaw0 "Ini yaw-angle VEHICLE wrt GLOBAL axis system [deg]"; wheelRadius "Wheel Radius [m]"; hcog "Dynamics: hCoG [m]"; b "Dynamics: b [m]"; TimeStep "Time Step [s]"
      mask help:
      | This block encapsulates the base Contact sensor.
      |
      | It takes input parameters from the PreScan 3D vehicle dynamics block and outputs contact results.
      mask Help: eval('openHelp(251)')
  SELF_Demux : Subsystem  Tag=demux/SelfPort  mask(PreScan Demux Block:){}
      mask help:
      | The SELF port shows (state) information of the actor itself. The outputs are position in the experiment's axis system and the GPS coordinates, and the object's absolute velocity and compass heading.
      |
      | For more information, please click Help.
      settings: DeleteFcn=PreScanBlockDeleteFcn;
      mask Help: eval('openHelp(462)')
      mask Display:
      | port_label('output',1,'x [m]')
      | port_label('output',2,'y [m]')
      | port_label('output',3,'z [m]','texmode','on')
      | port_label('output',4,'Rotx [deg]','texmode','on')
      | port_label('output',5,'Roty [deg]','texmode','on')
      | port_label('output',6,'Rotz [deg]','texmode','on')
      | port_label('output',7,'GPS lat [deg]','texmode','on')
      | port_label('output',8,'GPS long [deg]','texmode','on')
      | port_label('output',9,'GPS alt [m]','texmode','on')
      | port_label('output',10,'Velocity [m/s]')
      | port_label('output',11,'Heading [deg]')
      | port_label('output',12,'Yaw rate [deg/s]')
  STATE_Audi_A8_Sedan_2 : Subsystem  Tag=mux/StatePort  Priority=0  LoadFcn=load PrescanStateActuatorData  mask(PreScan Sink Block: State){x0=62.0152, y0=90.3976, z0=0.55, Roll0=0, Pitch0=0, Yaw0=0, TimeStep=1/200}
      mask prompts: x0 "Ini x-position VEHICLE wrt GLOBAL axis system [m]"; y0 "Ini y-position VEHICLE wrt GLOBAL axis system [m]"; z0 "Ini z-position VEHICLE wrt GLOBAL axis system [m]"; Roll0 "Ini roll-angle BODY wrt VEHICLE axis system [deg]"; Pitch0 "Ini pitch-angle BODY wrt VEHICLE axis system [deg]"; Yaw0 "Ini yaw-angle VEHICLE wrt GLOBAL axis system [deg]"; TimeStep "Auto-Assigned: Upload Period [s]"
      mask help:
      | The Actor State contains a vector signal of size (9x1), containing the following signals:
      |
      | -  Position                  (x,y,z)                                     [m]
      | -  Velocity                  (vx,vy,vz)                               [m/s]
      | -  Angles                    (Roll, Pitch, Yaw)                   [rad]
      |
      | The Actor state is defined in the global axis system.
      | The state is superponed on the Initial position defined in the GUI.
      |
      | For more information, please click Help.
      settings: DeleteFcn=PreScanBlockDeleteFcn;
      mask Help: eval('openHelp(222)')
      mask Display: image(imread('State.png'))
  STATE_Audi_A8_Sedan_2_rc : RateTransition  Tag=mux_rc/StatePort  OutPortSampleTimeOpt=Inherit
  Terminator_{1..13} (13 alike) : Terminator
  WheelDisplacement_Mux : Subsystem  Tag=mux/JointGroup  mask(JointGroup){}
      mask help:
      | The JointGroup allows to control several Joints in one go, as defined for this particular model.
      | For more information, look in the PreScan manual in the section "Model Preparation Tool" -> "Joint Groups"
      |
      | For more information on the Joints simulink interface, press Help.
      mask Help: eval('openHelp(254)')
  STATE_Audi_A8_Sedan_2_bus : Outport  Tag=outport/StatePort  OutDataTypeStr=Bus: PRESCAN_STATEACTUATORDATA  PortDimensions=1  SampleTime=2/200
  WheelL0_Audi_A8_Sedan_2 : Outport  Tag=outport/JointActuator  Port=2  OutDataTypeStr=Bus: PRESCAN_POSE_DATA  SampleTime=2/200
  WheelL1_Audi_A8_Sedan_2 : Outport  Tag=outport/JointActuator  Port=3  OutDataTypeStr=Bus: PRESCAN_POSE_DATA  SampleTime=2/200
  WheelR0_Audi_A8_Sedan_2 : Outport  Tag=outport/JointActuator  Port=4  OutDataTypeStr=Bus: PRESCAN_POSE_DATA  SampleTime=2/200
  WheelR1_Audi_A8_Sedan_2 : Outport  Tag=outport/JointActuator  Port=5  OutDataTypeStr=Bus: PRESCAN_POSE_DATA  SampleTime=2/200
  wires:
  STATE_Audi_A8_Sedan_2_rc/1 -> STATE_Audi_A8_Sedan_2_bus/1
  STATE_Audi_A8_Sedan_2/1(StateBus) -> STATE_Audi_A8_Sedan_2_rc/1
  SELF_Audi_A8_Sedan_2/1 -> SELF_Demux/1(SELF)
  WheelDisplacement_Mux/1(WheelL0_Audi_A8_Sedan_2) -> WheelL0_Audi_A8_Sedan_2/1
  WheelDisplacement_Mux/2(WheelL1_Audi_A8_Sedan_2) -> WheelL1_Audi_A8_Sedan_2/1
  WheelDisplacement_Mux/3(WheelR0_Audi_A8_Sedan_2) -> WheelR0_Audi_A8_Sedan_2/1
  WheelDisplacement_Mux/4(WheelR1_Audi_A8_Sedan_2) -> WheelR1_Audi_A8_Sedan_2/1
  JointGroup_WheelDisplacement_V2R/1(Rotation [rad]) -> WheelDisplacement_Mux/3(Rotation [rad])
  Auto_Gear/1 -> Dynamics_Simple_3D/6(Auto_GearShift)
  Dynamics_Simple_3D/8(ContactParams) -> PreScan_Contact_Sensor/1(ContactParams)
  PreScan_Contact_Sensor/1(Results) -> Dynamics_Simple_3D/8(TyreInfo_in)
  Dynamics_Simple_3D/2(Vx [m s-1]) -> JointGroup_WheelDisplacement_V2R/1(Velocity [m/s])
  Dynamics_Simple_3D/4(z_wheelFL_[m]) -> WheelDisplacement_Mux/4(zDisp FL [m])
  Dynamics_Simple_3D/5(z_wheelFR_[m]) -> WheelDisplacement_Mux/5(zDisp FR [m])
  Dynamics_Simple_3D/6(z_wheelRL_[m]) -> WheelDisplacement_Mux/6(zDisp RL [m])
  Dynamics_Simple_3D/7(z_wheelRR_[m]) -> WheelDisplacement_Mux/7(zDisp RR [m])
  Dynamics_Simple_3D/1(State) -> STATE_Audi_A8_Sedan_2/1(State)
  Ground_1/1 -> Dynamics_Simple_3D/1(DeltaSteer_[deg])
  Ground_2/1 -> Dynamics_Simple_3D/2(Throttle)
  Ground_3/1 -> Dynamics_Simple_3D/3(Brake)
  Ground_4/1 -> Dynamics_Simple_3D/4(Initial_Vx_[ms-1])
  Ground_5/1 -> Dynamics_Simple_3D/5(AutoManual_OnOff)
  Ground_6/1 -> Dynamics_Simple_3D/7(Manual_GearShift)
  Dynamics_Simple_3D/3(Perf_Params) -> Terminator_1/1
  Ground_7/1 -> PreScan_Contact_Sensor/2(Steer Angle Front [deg])
  Ground_8/1 -> PreScan_Contact_Sensor/3(Steer Angle Rear [deg])
  SELF_Demux/1(x [m]) -> Terminator_2/1
  SELF_Demux/2(y [m]) -> Terminator_3/1
  SELF_Demux/3(z [m]) -> Terminator_4/1
  SELF_Demux/4(rotx [deg]) -> Terminator_5/1
  SELF_Demux/5(roty [deg]) -> Terminator_6/1
  SELF_Demux/6(rotz [deg]) -> Terminator_7/1
  SELF_Demux/7(GPS lat [deg]) -> Terminator_8/1
  SELF_Demux/8(GPS long [deg]) -> Terminator_9/1
  SELF_Demux/9(GPS alt [m]) -> Terminator_10/1
  SELF_Demux/10(velocity [m/s]) -> Terminator_11/1
  SELF_Demux/11(heading [deg]) -> Terminator_12/1
  SELF_Demux/12(yaw rate [deg/s]) -> Terminator_13/1
  Ground_9/1 -> WheelDisplacement_Mux/1(Steering Angle Front [rad])
  Ground_10/1 -> WheelDisplacement_Mux/2(Steering Angle Rear [rad])

== system LMS_cs_2018/Audi_A8_Sedan_3 ==
  SELF_Audi_A8_Sedan_3 : Inport  Tag=inport/SelfPort  OutDataTypeStr=Bus: PRESCAN_SELFSENSORDATA  PortDimensions=1  SampleTime=2/200  BusOutputAsStruct=on
  Auto_Gear : Constant  Tag=AutoGear
  Dynamics_Simple_3D : Subsystem  Tag=Simple_Vehicle_Dynamics_3D  mask(PreScan Block: Simple Dynamics 3D){Migrate=on, TimeStep=1/200, ComputationMode=Continuous_Time}
      mask prompts: Migrate "Migrate. During migration this block will be replaced by a newer one."; TimeStep "Auto assigned: Time Step [s]"; ComputationMode "Computation mode:"
      mask help:
      | The Simple Dynamics Model is selected in the GUI to simulate vehicle dynamics behavior.
      |
      | The Simple Dynamics Model is completely open to the user. The parameters of this model can be set in the Simple Dynamics dialog in the GUI.
      |
      | For more information, please click Help.
      mask init:
      | p = SimpleDyn_pars;
      settings: DeleteFcn=PreScanBlockDeleteFcn;
      mask Help: eval('openHelp(260)')
      mask Display:
      | image(imread('SimpleDyn.png'))
      | port_label('input', 1, '{\delta}_S_t_ _e_e_r [deg]','texmode','on')
      | port_label('input', 2, 'Throttle [%]')
      | port_label('input', 3, 'Brake Pres [bar]')
      | port_label('input', 4, 'V_0 [ms-1]','texmode','on')
      | port_label('input', 5, 'Auto=[0]/Manual=[1]')
      | port_label('input', 6, 'Auto_GearShift')
      | port_label('input', 7, 'Manual_GearShift')
      | port_label('input', 8, 'TyreInfo_in')
      | port_label('output', 1, 'State')
      | port_label('output', 2, 'Vx [ms-1]')
      | port_label('output', 3, 'Perf Params')
      | port_label('output', 4, 'zDispFL[m]')
      | port_label('output', 5, 'zDispFR[m]')
      | port_label('output', 6, 'zDispRL[m]')
      | port_label('output', 7, 'zDispRR[m]')
  Ground_{1..10} (10 alike) : Ground
  JointGroup_WheelDisplacement_V2R : Subsystem  Tag=mux/Wheels  mask(PreScan Velocity to Wheel Angle Block:){TimeStep=2/200, TireRadius=0.34}
      mask prompts: TimeStep "Auto Assigned: Time Step [s]"; TireRadius "Tire Radius [m]"
      settings: DeleteFcn=PreScanBlockDeleteFcn;
      mask Display: disp('Velocity\nto\nWheelAngle')
  PreScan_Contact_Sensor : Subsystem  Tag=PreScan_Contact_Sensor  LoadFcn=|  mask(PreScan Block: PreScan Contact Sensor){x0=123.3257, y0=94.1389, z0=0.55, Roll0=0, Pitch0=0, Yaw0=0, wheelRadius=0.34, hcog=0.55, b=1.77, TimeStep=1/200}
      | load PrescanXYZData;
      | load PrescanRPYData;
      | load PrescanQuatData;
      | load PrescanAxisAngleData;
      | load PrescanPoseData;
      | load PrescanPoseQData;
      | load PrescanPoseAData;
      | load PrescanWheelContactData;
      mask prompts: x0 "Ini x-position VEHICLE wrt GLOBAL axis system [m]"; y0 "Ini y-position VEHICLE wrt GLOBAL axis system [m]"; z0 "Ini z-position VEHICLE wrt GLOBAL axis system [m]"; Roll0 "Ini roll-angle BODY wrt VEHICLE axis system [deg]"; Pitch0 "Ini pitch-angle BODY wrt VEHICLE axis system [deg]"; Yaw0 "Ini yaw-angle VEHICLE wrt GLOBAL axis system [deg]"; wheelRadius "Wheel Radius [m]"; hcog "Dynamics: hCoG [m]"; b "Dynamics: b [m]"; TimeStep "Time Step [s]"
      mask help:
      | This block encapsulates the base Contact sensor.
      |
      | It takes input parameters from the PreScan 3D vehicle dynamics block and outputs contact results.
      mask Help: eval('openHelp(251)')
  SELF_Demux : Subsystem  Tag=demux/SelfPort  mask(PreScan Demux Block:){}
      mask help:
      | The SELF port shows (state) information of the actor itself. The outputs are position in the experiment's axis system and the GPS coordinates, and the object's absolute velocity and compass heading.
      |
      | For more information, please click Help.
      settings: DeleteFcn=PreScanBlockDeleteFcn;
      mask Help: eval('openHelp(462)')
      mask Display:
      | port_label('output',1,'x [m]')
      | port_label('output',2,'y [m]')
      | port_label('output',3,'z [m]','texmode','on')
      | port_label('output',4,'Rotx [deg]','texmode','on')
      | port_label('output',5,'Roty [deg]','texmode','on')
      | port_label('output',6,'Rotz [deg]','texmode','on')
      | port_label('output',7,'GPS lat [deg]','texmode','on')
      | port_label('output',8,'GPS long [deg]','texmode','on')
      | port_label('output',9,'GPS alt [m]','texmode','on')
      | port_label('output',10,'Velocity [m/s]')
      | port_label('output',11,'Heading [deg]')
      | port_label('output',12,'Yaw rate [deg/s]')
  STATE_Audi_A8_Sedan_3 : Subsystem  Tag=mux/StatePort  Priority=0  LoadFcn=load PrescanStateActuatorData  mask(PreScan Sink Block: State){x0=123.3257, y0=94.1389, z0=0.55, Roll0=0, Pitch0=0, Yaw0=0, TimeStep=1/200}
      mask prompts: x0 "Ini x-position VEHICLE wrt GLOBAL axis system [m]"; y0 "Ini y-position VEHICLE wrt GLOBAL axis system [m]"; z0 "Ini z-position VEHICLE wrt GLOBAL axis system [m]"; Roll0 "Ini roll-angle BODY wrt VEHICLE axis system [deg]"; Pitch0 "Ini pitch-angle BODY wrt VEHICLE axis system [deg]"; Yaw0 "Ini yaw-angle VEHICLE wrt GLOBAL axis system [deg]"; TimeStep "Auto-Assigned: Upload Period [s]"
      mask help:
      | The Actor State contains a vector signal of size (9x1), containing the following signals:
      |
      | -  Position                  (x,y,z)                                     [m]
      | -  Velocity                  (vx,vy,vz)                               [m/s]
      | -  Angles                    (Roll, Pitch, Yaw)                   [rad]
      |
      | The Actor state is defined in the global axis system.
      | The state is superponed on the Initial position defined in the GUI.
      |
      | For more information, please click Help.
      settings: DeleteFcn=PreScanBlockDeleteFcn;
      mask Help: eval('openHelp(222)')
      mask Display: image(imread('State.png'))
  STATE_Audi_A8_Sedan_3_rc : RateTransition  Tag=mux_rc/StatePort  OutPortSampleTimeOpt=Inherit
  Terminator_{1..13} (13 alike) : Terminator
  WheelDisplacement_Mux : Subsystem  Tag=mux/JointGroup  mask(JointGroup){}
      mask help:
      | The JointGroup allows to control several Joints in one go, as defined for this particular model.
      | For more information, look in the PreScan manual in the section "Model Preparation Tool" -> "Joint Groups"
      |
      | For more information on the Joints simulink interface, press Help.
      mask Help: eval('openHelp(254)')
  STATE_Audi_A8_Sedan_3_bus : Outport  Tag=outport/StatePort  OutDataTypeStr=Bus: PRESCAN_STATEACTUATORDATA  PortDimensions=1  SampleTime=2/200
  WheelL0_Audi_A8_Sedan_3 : Outport  Tag=outport/JointActuator  Port=2  OutDataTypeStr=Bus: PRESCAN_POSE_DATA  SampleTime=2/200
  WheelL1_Audi_A8_Sedan_3 : Outport  Tag=outport/JointActuator  Port=3  OutDataTypeStr=Bus: PRESCAN_POSE_DATA  SampleTime=2/200
  WheelR0_Audi_A8_Sedan_3 : Outport  Tag=outport/JointActuator  Port=4  OutDataTypeStr=Bus: PRESCAN_POSE_DATA  SampleTime=2/200
  WheelR1_Audi_A8_Sedan_3 : Outport  Tag=outport/JointActuator  Port=5  OutDataTypeStr=Bus: PRESCAN_POSE_DATA  SampleTime=2/200
  wires:
  STATE_Audi_A8_Sedan_3_rc/1 -> STATE_Audi_A8_Sedan_3_bus/1
  STATE_Audi_A8_Sedan_3/1(StateBus) -> STATE_Audi_A8_Sedan_3_rc/1
  SELF_Audi_A8_Sedan_3/1 -> SELF_Demux/1(SELF)
  WheelDisplacement_Mux/1(WheelL0_Audi_A8_Sedan_3) -> WheelL0_Audi_A8_Sedan_3/1
  WheelDisplacement_Mux/2(WheelL1_Audi_A8_Sedan_3) -> WheelL1_Audi_A8_Sedan_3/1
  WheelDisplacement_Mux/3(WheelR0_Audi_A8_Sedan_3) -> WheelR0_Audi_A8_Sedan_3/1
  WheelDisplacement_Mux/4(WheelR1_Audi_A8_Sedan_3) -> WheelR1_Audi_A8_Sedan_3/1
  JointGroup_WheelDisplacement_V2R/1(Rotation [rad]) -> WheelDisplacement_Mux/3(Rotation [rad])
  Auto_Gear/1 -> Dynamics_Simple_3D/6(Auto_GearShift)
  Dynamics_Simple_3D/8(ContactParams) -> PreScan_Contact_Sensor/1(ContactParams)
  PreScan_Contact_Sensor/1(Results) -> Dynamics_Simple_3D/8(TyreInfo_in)
  Dynamics_Simple_3D/2(Vx [m s-1]) -> JointGroup_WheelDisplacement_V2R/1(Velocity [m/s])
  Dynamics_Simple_3D/4(z_wheelFL_[m]) -> WheelDisplacement_Mux/4(zDisp FL [m])
  Dynamics_Simple_3D/5(z_wheelFR_[m]) -> WheelDisplacement_Mux/5(zDisp FR [m])
  Dynamics_Simple_3D/6(z_wheelRL_[m]) -> WheelDisplacement_Mux/6(zDisp RL [m])
  Dynamics_Simple_3D/7(z_wheelRR_[m]) -> WheelDisplacement_Mux/7(zDisp RR [m])
  Dynamics_Simple_3D/1(State) -> STATE_Audi_A8_Sedan_3/1(State)
  Ground_1/1 -> Dynamics_Simple_3D/1(DeltaSteer_[deg])
  Ground_2/1 -> Dynamics_Simple_3D/2(Throttle)
  Ground_3/1 -> Dynamics_Simple_3D/3(Brake)
  Ground_4/1 -> Dynamics_Simple_3D/4(Initial_Vx_[ms-1])
  Ground_5/1 -> Dynamics_Simple_3D/5(AutoManual_OnOff)
  Ground_6/1 -> Dynamics_Simple_3D/7(Manual_GearShift)
  Dynamics_Simple_3D/3(Perf_Params) -> Terminator_1/1
  Ground_7/1 -> PreScan_Contact_Sensor/2(Steer Angle Front [deg])
  Ground_8/1 -> PreScan_Contact_Sensor/3(Steer Angle Rear [deg])
  SELF_Demux/1(x [m]) -> Terminator_2/1
  SELF_Demux/2(y [m]) -> Terminator_3/1
  SELF_Demux/3(z [m]) -> Terminator_4/1
  SELF_Demux/4(rotx [deg]) -> Terminator_5/1
  SELF_Demux/5(roty [deg]) -> Terminator_6/1
  SELF_Demux/6(rotz [deg]) -> Terminator_7/1
  SELF_Demux/7(GPS lat [deg]) -> Terminator_8/1
  SELF_Demux/8(GPS long [deg]) -> Terminator_9/1
  SELF_Demux/9(GPS alt [m]) -> Terminator_10/1
  SELF_Demux/10(velocity [m/s]) -> Terminator_11/1
  SELF_Demux/11(heading [deg]) -> Terminator_12/1
  SELF_Demux/12(yaw rate [deg/s]) -> Terminator_13/1
  Ground_9/1 -> WheelDisplacement_Mux/1(Steering Angle Front [rad])
  Ground_10/1 -> WheelDisplacement_Mux/2(Steering Angle Rear [rad])
